simulink model "sin_compensar_discreto"  (R2015a)
settings: Solver=ode45  StartTime=0.0  StopTime=10  RelTol=1e-3
undefined symbols (not defined in the file): Bm, DisAng, Ga, Gb, Jt, Kb, Ki, L, PosInicial, R, RelacionEngranajes, Rrueda
libraries: simulink x1
settings Model: Creator=familia colazo  LastModifiedBy=familia colazo

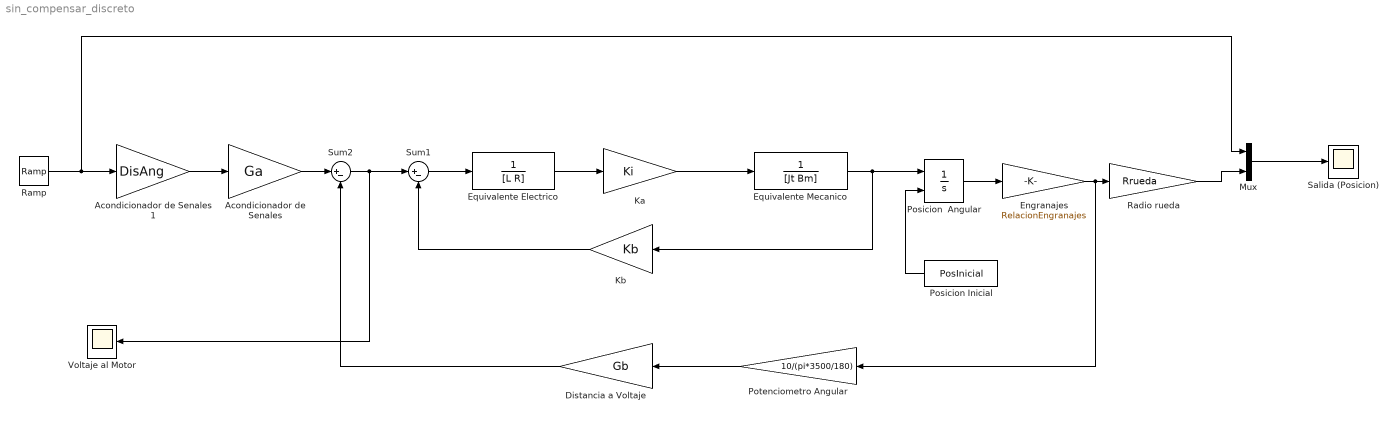
== system sin_compensar_discreto ==
  "Acondicionador de Senales " : Gain  Gain=Ga
  Acondicionador de Senales 1 : Gain  Gain=DisAng
  Distancia a Voltaje : Gain  Gain=Gb
  "Engranajes " : Gain  Gain=RelacionEngranajes
  Equivalente Electrico : TransferFcn  Denominator=[L R]
  Equivalente Mecanico : TransferFcn  Denominator=[Jt Bm]
  Ka : Gain  Gain=Ki
  Kb : Gain  Gain=Kb
  Mux : Mux  Inputs=2
  Posicion  Angular : Integrator  InitialConditionSource=external
  Posicion Inicial : Constant  Value=PosInicial
  "Potenciometro Angular " : Gain  Gain=10/(pi*3500/180)
  Radio rueda : Gain  Gain=Rrueda
  Ramp : simulink/Sources/Ramp  slope=1  start=0  X0=0
  Salida (Posicion) : Scope
      settings: TickLabels=on  TimeRange=14  YMin=-0.751036  YMax=0.0612263  SampleInput=on
  Sum1 : Sum  Inputs=|+-
  Sum2 : Sum  Inputs=|+-
  Voltaje al Motor : Scope
      settings: TickLabels=on  TimeRange=14  YMin=-0.751036  YMax=0.0612263  SaveName=ScopeData2  SampleInput=on
  wires:
  Mux/1 -> Salida (Posicion)/1
  Ramp/1 -> Mux/1, Acondicionador de Senales 1/1
  Distancia a Voltaje/1 -> Sum2/2
  Posicion Inicial/1 -> Posicion  Angular/2
  Sum2/1 -> Sum1/1, Voltaje al Motor/1
  Kb/1 -> Sum1/2
  Equivalente Mecanico/1 -> Kb/1, Posicion  Angular/1
  Equivalente Electrico/1 -> Ka/1
  Sum1/1 -> Equivalente Electrico/1
  Ka/1 -> Equivalente Mecanico/1
  "Engranajes "/1 -> "Potenciometro Angular "/1, Radio rueda/1
  "Acondicionador de Senales "/1 -> Sum2/1
  Radio rueda/1 -> Mux/2
  Posicion  Angular/1 -> "Engranajes "/1
  "Potenciometro Angular "/1 -> Distancia a Voltaje/1
  Acondicionador de Senales 1/1 -> "Acondicionador de Senales "/1
